simulink model "car_model"  (R2022a)
settings: Solver=VariableStepAuto  StartTime=0.0  StopTime=10.0  RelTol=1e-3
undefined symbols (not defined in the file or in its folder): Iw
settings Model: Creator=sahil  LastModifiedBy=sahil

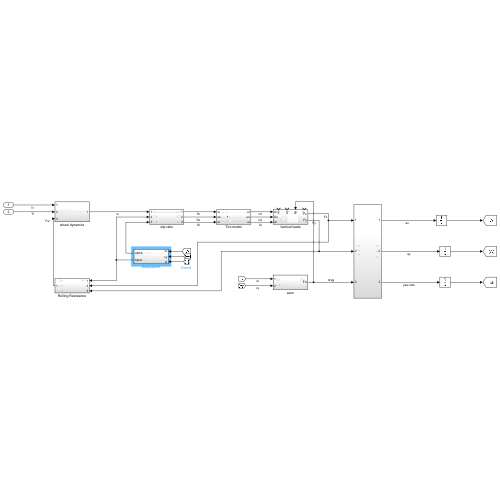
[thumbnail: Simulink's stored preview of the top-level diagram]
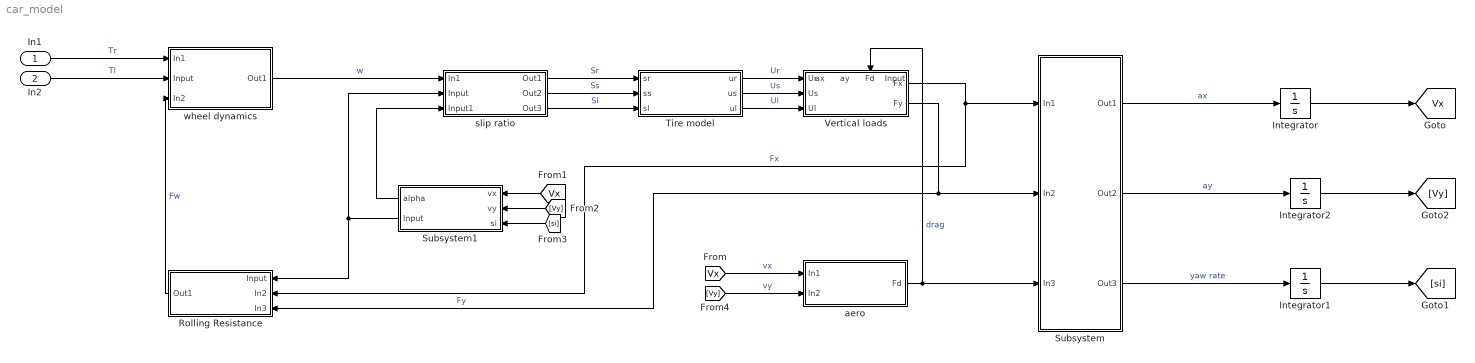
== system car_model ==
  In1 : Inport
  In2 : Inport  Port=2
  Integrator : Integrator
  Integrator1 : Integrator
  Integrator2 : Integrator
  Rolling Resistance : Subsystem
  Subsystem : Subsystem
  Subsystem1 : Subsystem
  Tire model : Subsystem
  Vertical loads : Subsystem
      settings: PortSchema="{\"entries\":[{\"content\":{\"sides\":[{\"content\":{\"connectorIds\":[\"In1\",\"In2\",\"In3\"]},\"type\":\"ConnectorPlacement.EquallySpacedRectSide\",\"uuid\":\"c87bc92c-d52c-4e2b-afec-a565792782b9\"},{\"content\":{\"connectorIds\":[\"Out1\",\"Out2\"],\"side\":\"RIGHT\"},\"type\":\"ConnectorPlacement.EquallySpacedRectSide\",\"uuid\":\"3567d5cd-158a-4938-8187-fe829b738e45\"},{\"content\":{\"connectorIds\":[\"In4\",\"In5\",\"In6\",\"In7\"],\"side\":\"TOP\"},\"type\":\"ConnectorPlacement.EquallySpacedRectSide\",\"uuid\":\"f06ac3c6-4966-445b-b456-5d7cafdea9cf\"}]},\"type\":\"ConnectorPlacement.EquallySpacedConnector\",\"uuid\":\"42a630f0-6c67-471b-ab2b-99a4df149645\"}],\"packageUris\":[\"http://schema.mathworks.com/mf0/Connector/R2020b\"],\"version\":\"1.0\"}"
  aero : Subsystem
  slip ratio : Subsystem
  wheel dynamics : Subsystem
  tag scope: Vx=global
  wires:
  In1/1 -> wheel dynamics/1(In1)  "Tr"
  In2/1 -> wheel dynamics/2(Input)  "Tl"
  wheel dynamics/1(Out1) -> slip ratio/1(In1)  "w"
  slip ratio/1(Out1) -> Tire model/1(sr)  "Sr"
  slip ratio/2(Out2) -> Tire model/2(ss)  "Ss"
  slip ratio/3(Out3) -> Tire model/3(sl)  "Sl"
  Tire model/2(us) -> Vertical loads/2(Us)  "Us"
  Tire model/1(ur) -> Vertical loads/1(Ur)  "Ur"
  Tire model/3(ul) -> Vertical loads/3(Ul)  "Ul"
  Rolling Resistance/1(Out1) -> wheel dynamics/3(In2)  "Fw"
  Vertical loads/1(Fx) -> Rolling Resistance/2(In2), Subsystem/1(In1)  "Fx"
  Vertical loads/2(Fy) -> Rolling Resistance/3(In3), Subsystem/2(In2)  "Fy"
  aero/1(Fd) -> Subsystem/3(In3), Vertical loads/6(Fd)  "drag"
  [Vx] -> aero/1(In1)  "vx"
  [Vy] -> aero/2(In2)  "vy"
  Subsystem/1(Out1) -> Integrator/1  "ax"
  Subsystem/2(Out2) -> Integrator2/1  "ay"
  Subsystem/3(Out3) -> Integrator1/1  "yaw rate"
  Subsystem1/1(alpha) -> slip ratio/3(Input1)
  Subsystem1/2(Input) -> Rolling Resistance/1(Input), slip ratio/2(Input)
  Integrator/1 -> [Vx]
  Integrator2/1 -> [Vy]
  Integrator1/1 -> [si]
  [Vx] -> Subsystem1/1(vx)
  [Vy] -> Subsystem1/2(vy)
  [si] -> Subsystem1/3(si)

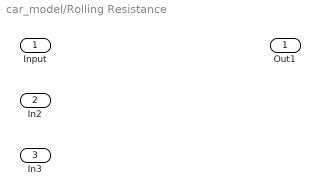
== system car_model/Rolling Resistance ==
  Input : Inport
  In2 : Inport  Port=2
  In3 : Inport  Port=3
  Out1 : Outport

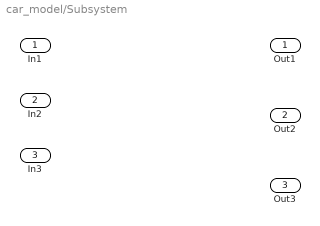
== system car_model/Subsystem ==
  In1 : Inport
  In2 : Inport  Port=2
  In3 : Inport  Port=3
  Out1 : Outport
  Out2 : Outport  Port=2
  Out3 : Outport  Port=3

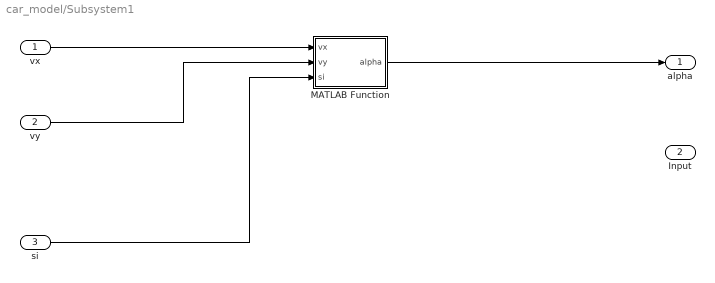
== system car_model/Subsystem1 ==
  vx : Inport
  vy : Inport  Port=2
  si : Inport  Port=3
  MATLAB Function : MATLAB Function  TreatAsAtomicUnit=on
  alpha : Outport
  Input : Outport  Port=2
  wires:
  vx/1 -> MATLAB Function/1(vx)
  vy/1 -> MATLAB Function/2(vy)
  si/1 -> MATLAB Function/3(si)
  MATLAB Function/1(alpha) -> alpha/1

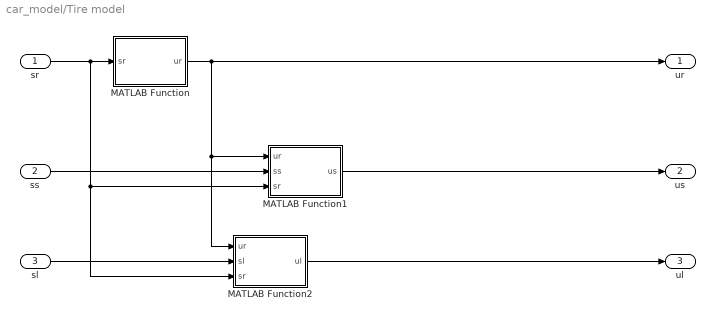
== system car_model/Tire model ==
  sr : Inport
  ss : Inport  Port=2
  sl : Inport  Port=3
  MATLAB Function : MATLAB Function  TreatAsAtomicUnit=on
  MATLAB Function1 : MATLAB Function  TreatAsAtomicUnit=on
  MATLAB Function2 : MATLAB Function  TreatAsAtomicUnit=on
  ur : Outport
  us : Outport  Port=2
  ul : Outport  Port=3
  wires:
  sr/1 -> MATLAB Function2/3(sr), MATLAB Function1/3(sr), MATLAB Function/1(sr)
  MATLAB Function/1(ur) -> ur/1, MATLAB Function2/1(ur), MATLAB Function1/1(ur)
  ss/1 -> MATLAB Function1/2(ss)
  MATLAB Function1/1(us) -> us/1
  sl/1 -> MATLAB Function2/2(sl)
  MATLAB Function2/1(ul) -> ul/1

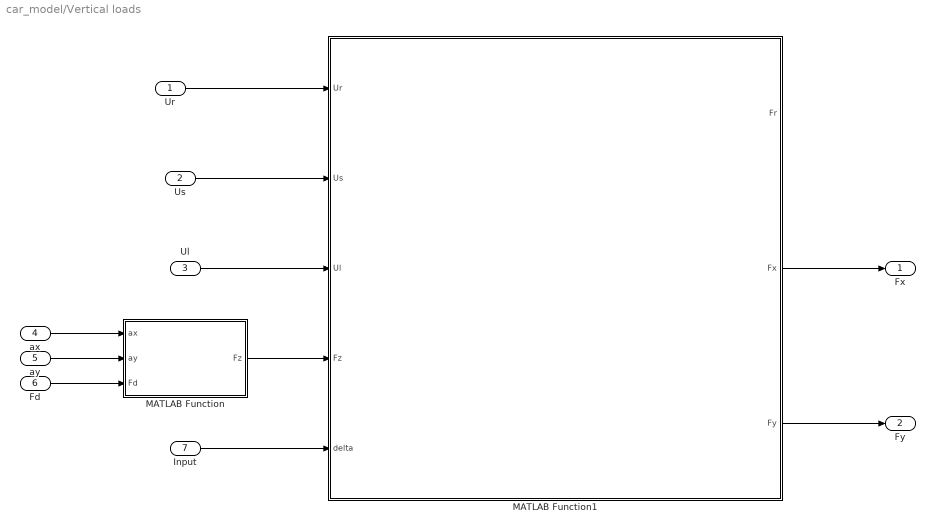
== system car_model/Vertical loads ==
  Ur : Inport
  Us : Inport  Port=2
  Ul : Inport  Port=3
  ax : Inport  Port=4
  ay : Inport  Port=5
  Fd : Inport  Port=6
  Input : Inport  Port=7
  MATLAB Function : MATLAB Function  TreatAsAtomicUnit=on
  MATLAB Function1 : MATLAB Function  TreatAsAtomicUnit=on
  Fx : Outport
  Fy : Outport  Port=2
  wires:
  ay/1 -> MATLAB Function/2(ay)
  ax/1 -> MATLAB Function/1(ax)
  Fd/1 -> MATLAB Function/3(Fd)
  Ul/1 -> MATLAB Function1/3(Ul)
  Us/1 -> MATLAB Function1/2(Us)
  Ur/1 -> MATLAB Function1/1(Ur)
  MATLAB Function/1(Fz) -> MATLAB Function1/4(Fz)
  MATLAB Function1/2(Fx) -> Fx/1
  MATLAB Function1/3(Fy) -> Fy/1
  Input/1 -> MATLAB Function1/5(delta)

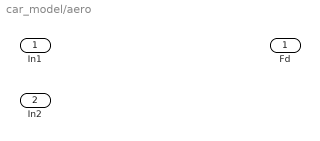
== system car_model/aero ==
  In1 : Inport
  In2 : Inport  Port=2
  Fd : Outport

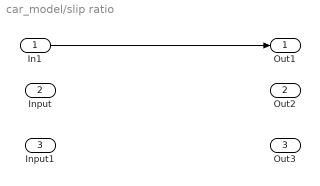
== system car_model/slip ratio ==
  In1 : Inport
  Input : Inport  Port=2
  Input1 : Inport  Port=3
  Out1 : Outport
  Out2 : Outport  Port=2
  Out3 : Outport  Port=3
  wires:
  In1/1 -> Out1/1

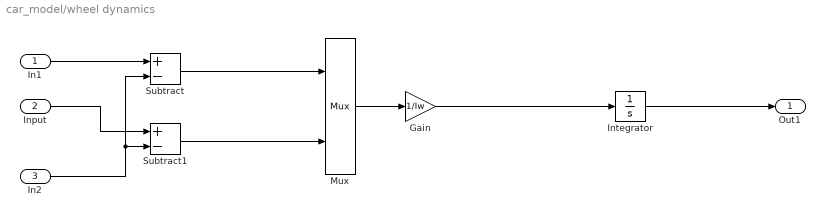
== system car_model/wheel dynamics ==
  In1 : Inport
  Input : Inport  Port=2
  In2 : Inport  Port=3
  Gain : Gain  Gain=1/Iw
  Integrator : Integrator
  Mux : Mux  Inputs=2
  Subtract : Sum  Inputs=+-
  Subtract1 : Sum  Inputs=+-
  Out1 : Outport
  wires:
  Input/1 -> Subtract1/1
  In2/1 -> Subtract/2, Subtract1/2
  In1/1 -> Subtract/1
  Subtract/1 -> Mux/1
  Subtract1/1 -> Mux/2
  Mux/1 -> Gain/1
  Gain/1 -> Integrator/1
  Integrator/1 -> Out1/1

== matlab function car_model/Tire model/MATLAB Function1 ==
  data: ur input; us output; ss input; sr input
function us = fcn(ur , ss , sr)
    us=ur.*(ss./sr);

== matlab function car_model/Tire model/MATLAB Function ==
  data: sr input; ur output
function ur = fcn(sr)
C1=1;
C2=1;
C3=1;



ur = C1*(1-exp(-C2*sr))-C3*sr;

== matlab function car_model/Tire model/MATLAB Function2 ==
  data: ur input; ul output; sl input; sr input
function ul = fcn(ur , sl , sr)
    ul=ur.*(sl./sr);

== matlab function car_model/Vertical loads/MATLAB Function ==
  data: ax input; Fz output; ay input; Fd input
function Fz = fcn(ax,ay,Fd)
 hcg=1;
 hd=1;
 wf=1;
 wr=1;
 twf=1;
 twr=1;
 g=9.81;
 m=229;
 Fzr= m*g*wf/(wf+wr)+(Fd*hd+m*ax*hcg)/(wf+wr);
 Fzf= m*g*wr/(wf+wr)-(Fd*hd+m*ax*hcg)/(wf+wr);
 Fzfl= (Fzf/2)*(twf/2)+ay*hcg*Fzf/g;
 Fzfr= (Fzf/2)*(twf/2)-ay*hcg*Fzf/g;
 Fzrl=(Fzr/2)*(twr/2)+ay*hcg*Fzr/g;
 Fzrr=(Fzr/2)*(twr/2)-ay*hcg*Fzr/g;
 Fz=[Fzfl Fzfr; Fzrl Fzrr];

== matlab function car_model/Vertical loads/MATLAB Function1 ==
  data: Ur input; Us input; Ul input; Fr output; Fz input; Fx output; Fy output; delta input
function [Fr,Fx,Fy] = fcn(Ur,Us,Ul,Fz, delta)

Q=[cos(delta) sin(delta); -sin(delta) cos(delta)];
Fr = Ur.*Fz;
Fx1=Ul.*Fz;
Fy1=Us.*Fz;
Ff=magic(4);
Ff(1:2,1)=Transpose(Fx1(1,1:2));
Ff(1:2,2)=transpose(Fy1(1,1:2));
Ff1=Ff*Q;
Fx1(1,1:2)=transpose(Ff1(1:2,1));
Fy1(1,1:2)=transpose(Ff2(1:2,2));
Fx=sum(Fx1,"all");
Fy=sum(Fy1,"all");

== matlab function car_model/Subsystem1/MATLAB Function ==
  data: vx input; alpha output; vy input; si input
function alpha = fcn(vx,vy,si)
xi=[wbf wbf; -wbr -wbr];
yi=tw/2*[1 -1; 1 -1];
ratio=atan((vy+xi*si)./(vx-yi*si));
alpha=ratio-delta;
